simulink model "DKver1"  (R2013b)
settings: Solver=ode45  StartTime=0.0  StopTime=20000.0  RelTol=1e-3
libraries: xbsIndex_r4 x132, dspsrcs4 x4
settings Model: Creator=Robot  LastModifiedBy=Robot32-VM

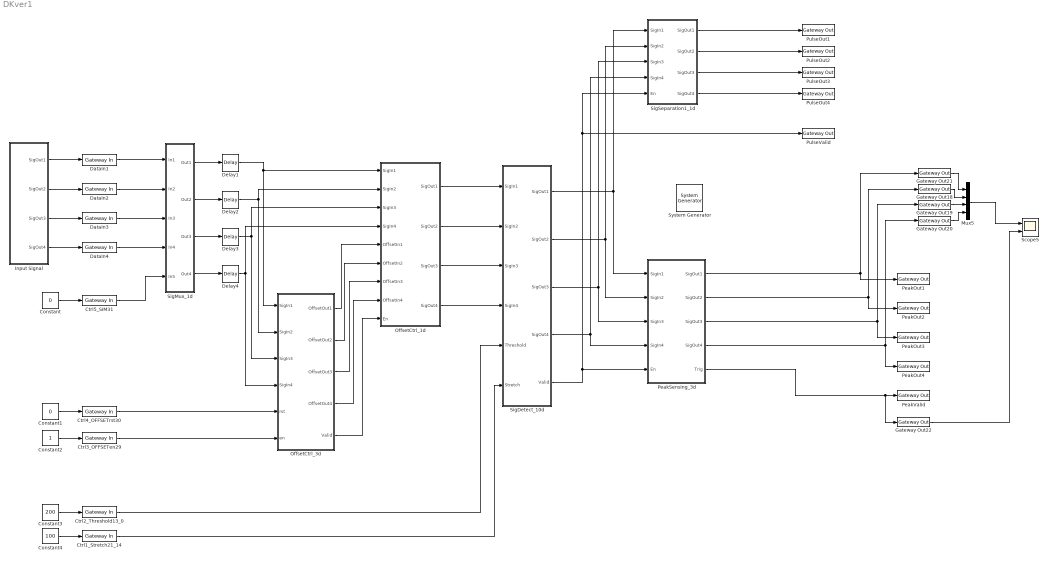
== system DKver1 ==
  " System Generator" : xbsIndex_r4/ System Generator  Tag=genX  xilinxfamily=spartan6  part=xc6slx45  speed=-2  package=fgg484  synthesis_tool=XST  clock_wrapper=Clock Enables  directory=C:/Users/Robot32-VM/Documents/System Generator/11_Gamma_Simple/1_HDL_Netlist_lx45  proj_type=Project Navigator  Synth_file=XST Defaults  Impl_file=ISE Defaults  testbench=off  simulink_period=1  sysclk_period=9  dcm_input_clock_period=10  incr_netlist=off  trim_vbits=Everywhere in SubSystem  dbl_ovrd=According to Block Masks  core_generation=According to Block Masks  run_coregen=off  deprecated_control=off  eval_field=0  block_type=sysgen
  Constant : Constant  Value=0
  Constant1 : Constant  Value=0
  Constant2 : Constant
  Constant3 : Constant  Value=200
  Constant4 : Constant  Value=100
  Ctrl1_Stretch21_14 : xbsIndex_r4/Gateway In  gui_display_data_type=Fixed-point  arith_type=Unsigned  n_bits=8  bin_pt=0  preci_type=Single  exp_width=8  frac_width=24  quantization="Round  (unbiased: +/- Inf)"  overflow=Saturate  period=1  dbl_ovrd=off  timing_constraint=None  locs_specified=off  LOCs={}  UseAsADC=off  ADCChannel='1'  inherit_from_input=off  hdl_port=on  block_type=gatewayin
  Ctrl2_Threshold13_0 : xbsIndex_r4/Gateway In  gui_display_data_type=Fixed-point  arith_type="Signed  (2's comp)"  n_bits=14  bin_pt=0  preci_type=Single  exp_width=8  frac_width=24  quantization="Round  (unbiased: +/- Inf)"  overflow=Saturate  period=1  dbl_ovrd=off  timing_constraint=None  locs_specified=off  LOCs={}  UseAsADC=off  ADCChannel='1'  inherit_from_input=off  hdl_port=on  block_type=gatewayin
  Ctrl3_OFFSETen29 : xbsIndex_r4/Gateway In  gui_display_data_type=Boolean  arith_type=Boolean  n_bits=16  bin_pt=14  preci_type=Single  exp_width=8  frac_width=24  quantization="Round  (unbiased: +/- Inf)"  overflow=Saturate  period=1  dbl_ovrd=off  timing_constraint=None  locs_specified=off  LOCs={}  UseAsADC=off  ADCChannel='1'  inherit_from_input=off  hdl_port=on  block_type=gatewayin
  Ctrl4_OFFSETrst30 : xbsIndex_r4/Gateway In  gui_display_data_type=Boolean  arith_type=Boolean  n_bits=16  bin_pt=14  preci_type=Single  exp_width=8  frac_width=24  quantization="Round  (unbiased: +/- Inf)"  overflow=Saturate  period=1  dbl_ovrd=off  timing_constraint=None  locs_specified=off  LOCs={}  UseAsADC=off  ADCChannel='1'  inherit_from_input=off  hdl_port=on  block_type=gatewayin
  Ctrl5_SIM31 : xbsIndex_r4/Gateway In  gui_display_data_type=Boolean  arith_type=Boolean  n_bits=16  bin_pt=14  preci_type=Single  exp_width=8  frac_width=24  quantization="Round  (unbiased: +/- Inf)"  overflow=Saturate  period=1  dbl_ovrd=off  timing_constraint=None  locs_specified=off  LOCs={}  UseAsADC=off  ADCChannel='1'  inherit_from_input=off  hdl_port=on  block_type=gatewayin
  DataIn{1..4} (4 alike) : xbsIndex_r4/Gateway In  gui_display_data_type=Fixed-point  arith_type="Signed  (2's comp)"  n_bits=14  bin_pt=0  preci_type=Single  exp_width=8  frac_width=24  quantization="Round  (unbiased: +/- Inf)"  overflow=Saturate  period=1  dbl_ovrd=off  timing_constraint=None  locs_specified=off  LOCs={}  UseAsADC=off  ADCChannel='1'  inherit_from_input=off  hdl_port=on  block_type=gatewayin
  Delay{1..4} (4 alike) : xbsIndex_r4/Delay  rst=off  infoeditControl=Selection of Reset will increase slice count due to use of real FFs and instead of SRLs  en=off  latency=1  dbl_ovrd=off  reg_retiming=off  block_type=delay
  Gateway Out{18..22} (5 alike) : xbsIndex_r4/Gateway Out  inherit_from_input=off  hdl_port=off  timing_constraint=None  locs_specified=off  LOCs={}  UseAsDAC=off  DACChannel='1'  block_type=gatewayout
  Input Signal : Subsystem
  Mux5 : Mux
  OffsetCtrl_1d : Subsystem
  OffsetCtrl_3d : Subsystem
  PeakOut{1..4} (4 alike) : xbsIndex_r4/Gateway Out  inherit_from_input=off  hdl_port=on  timing_constraint=None  locs_specified=off  LOCs={}  UseAsDAC=off  DACChannel='1'  block_type=gatewayout
  PeakSensing_3d : Subsystem
  PeakValid : xbsIndex_r4/Gateway Out  inherit_from_input=off  hdl_port=on  timing_constraint=None  locs_specified=off  LOCs={}  UseAsDAC=off  DACChannel='1'  block_type=gatewayout
  PulseOut{1..4} (4 alike) : xbsIndex_r4/Gateway Out  inherit_from_input=off  hdl_port=on  timing_constraint=None  locs_specified=off  LOCs={}  UseAsDAC=off  DACChannel='1'  block_type=gatewayout
  PulseValid : xbsIndex_r4/Gateway Out  inherit_from_input=off  hdl_port=on  timing_constraint=None  locs_specified=off  LOCs={}  UseAsDAC=off  DACChannel='1'  block_type=gatewayout
  Scope5 : Scope  NumInputPorts=2
      settings: YMin=-5~-5  YMax=5~5  SaveName=ScopeData8
  SigDetect_10d : Subsystem
  SigMux_1d : Subsystem
  SigSeparation1_1d : Subsystem
  wires:
  Input Signal/1(SigOut1) -> DataIn1/1
  Input Signal/2(SigOut2) -> DataIn2/1
  Input Signal/3(SigOut3) -> DataIn3/1
  Input Signal/4(SigOut4) -> DataIn4/1
  Constant/1 -> Ctrl5_SIM31/1
  Constant1/1 -> Ctrl4_OFFSETrst30/1
  Constant2/1 -> Ctrl3_OFFSETen29/1
  Constant3/1 -> Ctrl2_Threshold13_0/1
  Constant4/1 -> Ctrl1_Stretch21_14/1
  DataIn1/1 -> SigMux_1d/1(In1)
  DataIn2/1 -> SigMux_1d/2(In2)
  DataIn3/1 -> SigMux_1d/3(In3)
  DataIn4/1 -> SigMux_1d/4(In4)
  Ctrl5_SIM31/1 -> SigMux_1d/5(In5)
  SigMux_1d/1(Out1) -> Delay1/1
  SigMux_1d/2(Out2) -> Delay2/1
  SigMux_1d/3(Out3) -> Delay3/1
  SigMux_1d/4(Out4) -> Delay4/1
  Delay1/1 -> OffsetCtrl_3d/1(SigIn1), OffsetCtrl_1d/1(SigIn1)
  Delay2/1 -> OffsetCtrl_3d/2(SigIn2), OffsetCtrl_1d/2(SigIn2)
  Delay3/1 -> OffsetCtrl_1d/3(SigIn3), OffsetCtrl_3d/3(SigIn3)
  Delay4/1 -> OffsetCtrl_1d/4(SigIn4), OffsetCtrl_3d/4(SigIn4)
  Ctrl4_OFFSETrst30/1 -> OffsetCtrl_3d/5(rst)
  Ctrl3_OFFSETen29/1 -> OffsetCtrl_3d/6(en)
  OffsetCtrl_3d/1(OffsetOut1) -> OffsetCtrl_1d/5(OffsetIn1)
  OffsetCtrl_3d/2(OffsetOut2) -> OffsetCtrl_1d/6(OffsetIn2)
  OffsetCtrl_3d/3(OffsetOut3) -> OffsetCtrl_1d/7(OffsetIn3)
  OffsetCtrl_3d/4(OffsetOut4) -> OffsetCtrl_1d/8(OffsetIn4)
  OffsetCtrl_3d/5(Valid) -> OffsetCtrl_1d/9(En)
  OffsetCtrl_1d/1(SigOut1) -> SigDetect_10d/1(SigIn1)
  OffsetCtrl_1d/2(SigOut2) -> SigDetect_10d/2(SigIn2)
  OffsetCtrl_1d/3(SigOut3) -> SigDetect_10d/3(SigIn3)
  OffsetCtrl_1d/4(SigOut4) -> SigDetect_10d/4(SigIn4)
  Ctrl2_Threshold13_0/1 -> SigDetect_10d/5(Threshold)
  Ctrl1_Stretch21_14/1 -> SigDetect_10d/6(Stretch)
  SigSeparation1_1d/1(SigOut1) -> PulseOut1/1
  SigSeparation1_1d/2(SigOut2) -> PulseOut2/1
  SigSeparation1_1d/3(SigOut3) -> PulseOut3/1
  SigSeparation1_1d/4(SigOut4) -> PulseOut4/1
  SigDetect_10d/1(SigOut1) -> PeakSensing_3d/1(SigIn1), SigSeparation1_1d/1(SigIn1)
  SigDetect_10d/2(SigOut2) -> PeakSensing_3d/2(SigIn2), SigSeparation1_1d/2(SigIn2)
  SigDetect_10d/3(SigOut3) -> PeakSensing_3d/3(SigIn3), SigSeparation1_1d/3(SigIn3)
  SigDetect_10d/4(SigOut4) -> PeakSensing_3d/4(SigIn4), SigSeparation1_1d/4(SigIn4)
  PeakSensing_3d/5(Trig) -> Gateway Out22/1, PeakValid/1
  Mux5/1 -> Scope5/1
  Gateway Out21/1 -> Mux5/1
  Gateway Out18/1 -> Mux5/2
  Gateway Out19/1 -> Mux5/3
  Gateway Out20/1 -> Mux5/4
  Gateway Out22/1 -> Scope5/2
  PeakSensing_3d/1(SigOut1) -> PeakOut1/1, Gateway Out21/1
  PeakSensing_3d/2(SigOut2) -> PeakOut2/1, Gateway Out18/1
  PeakSensing_3d/3(SigOut3) -> PeakOut3/1, Gateway Out19/1
  PeakSensing_3d/4(SigOut4) -> PeakOut4/1, Gateway Out20/1
  SigDetect_10d/5(Valid) -> PulseValid/1, SigSeparation1_1d/5(En), PeakSensing_3d/5(En)

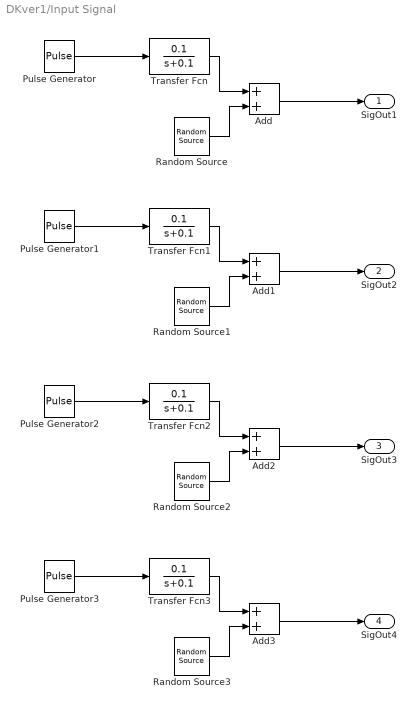
== system DKver1/Input Signal ==
  Add{,1..3} (4 alike) : Sum
  Pulse Generator : DiscretePulseGenerator  PulseType=Time based  Amplitude=5000  Period=1000
  Pulse Generator1 : DiscretePulseGenerator  PulseType=Time based  Amplitude=3000  Period=1000  PulseWidth=2  PhaseDelay=2
  Pulse Generator2 : DiscretePulseGenerator  PulseType=Time based  Amplitude=1000  Period=1000  PulseWidth=2  PhaseDelay=4
  Pulse Generator3 : DiscretePulseGenerator  PulseType=Time based  Amplitude=800  Period=1000  PulseWidth=2  PhaseDelay=6
  Random Source{,1..3} (4 alike) : dspsrcs4/Random Source  SrcType=Uniform  NormMethod=Ziggurat  CltLength=12  MinVal=-100  MaxVal=100  MeanVal=0  VarVal=1  RepMode=Not repeatable  rawSeed=1  IsInherit=off  SampMode=Discrete  SampTime=1  SampFrame=1  DataType=Double  OutComplex=Real
  Transfer Fcn{,1..3} (4 alike) : TransferFcn  Numerator=[0.1]  Denominator=[1 0.1]
  SigOut1 : Outport
  SigOut2 : Outport  Port=2
  SigOut3 : Outport  Port=3
  SigOut4 : Outport  Port=4
  wires:
  Add2/1 -> SigOut3/1
  Add1/1 -> SigOut2/1
  Add3/1 -> SigOut4/1
  Add/1 -> SigOut1/1
  Pulse Generator1/1 -> Transfer Fcn1/1
  Random Source/1 -> Add/2
  Transfer Fcn1/1 -> Add1/1
  Transfer Fcn2/1 -> Add2/1
  Random Source2/1 -> Add2/2
  Transfer Fcn3/1 -> Add3/1
  Pulse Generator3/1 -> Transfer Fcn3/1
  Random Source3/1 -> Add3/2
  Random Source1/1 -> Add1/2
  Pulse Generator2/1 -> Transfer Fcn2/1
  Transfer Fcn/1 -> Add/1
  Pulse Generator/1 -> Transfer Fcn/1

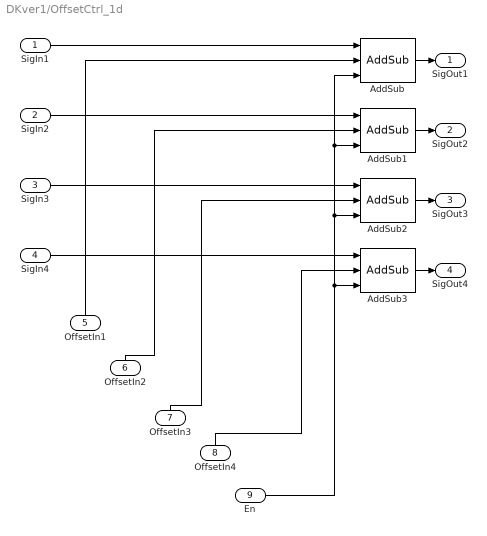
== system DKver1/OffsetCtrl_1d ==
  SigIn1 : Inport
  SigIn2 : Inport  Port=2
  SigIn3 : Inport  Port=3
  SigIn4 : Inport  Port=4
  OffsetIn1 : Inport  Port=5
  OffsetIn2 : Inport  Port=6
  OffsetIn3 : Inport  Port=7
  OffsetIn4 : Inport  Port=8
  En : Inport  Port=9
  AddSub{,1..3} (4 alike) : xbsIndex_r4/AddSub  mode=Subtraction  use_carryin=off  use_carryout=off  en=on  latency=1  precision=User Defined  arith_type="Signed  (2's comp)"  n_bits=14  bin_pt=0  quantization="Round  (unbiased: +/- Inf)"  overflow=Saturate  dbl_ovrd=off  use_behavioral_HDL=off  hw_selection=Fabric  pipelined=off  block_type=addsub
  SigOut1 : Outport
  SigOut2 : Outport  Port=2
  SigOut3 : Outport  Port=3
  SigOut4 : Outport  Port=4
  wires:
  OffsetIn1/1 -> AddSub/2
  SigIn4/1 -> AddSub3/1
  AddSub3/1 -> SigOut4/1
  En/1 -> AddSub3/3, AddSub2/3, AddSub1/3, AddSub/3
  SigIn2/1 -> AddSub1/1
  AddSub/1 -> SigOut1/1
  OffsetIn3/1 -> AddSub2/2
  AddSub1/1 -> SigOut2/1
  OffsetIn4/1 -> AddSub3/2
  AddSub2/1 -> SigOut3/1
  SigIn3/1 -> AddSub2/1
  SigIn1/1 -> AddSub/1
  OffsetIn2/1 -> AddSub1/2

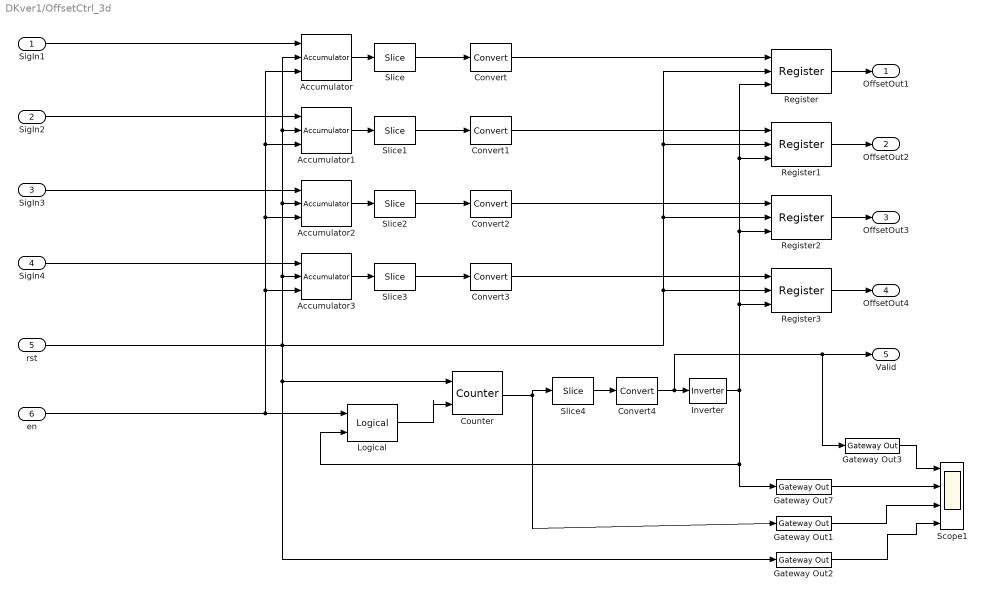
== system DKver1/OffsetCtrl_3d ==
  SigIn1 : Inport
  SigIn2 : Inport  Port=2
  SigIn3 : Inport  Port=3
  SigIn4 : Inport  Port=4
  rst : Inport  Port=5
  en : Inport  Port=6
  Accumulator{,1..3} (4 alike) : xbsIndex_r4/Accumulator  operation=Add  n_bits=32  overflow=Wrap  scale=1  rst=on  infoeditControl=reset for floating point data type must be asserted for a minimum of 2 cycles  hasbypass=off  en=on  latency=0  dbl_ovrd=off  msb_inp=100  msb=100  lsb=-100  use_behavioral_HDL=on  implementation=Fabric  block_type=accum
  Convert{,1..3} (4 alike) : xbsIndex_r4/Convert  gui_display_data_type=Fixed-point  arith_type="Signed  (2's comp)"  n_bits=20  bin_pt=0  float_type=Single  exp_bits=8  fraction_bits=24  quantization="Round  (unbiased: +/- Inf)"  overflow=Wrap  en=off  latency=1  dbl_ovrd=off  pipeline=off  block_type=convert
  Convert4 : xbsIndex_r4/Convert  gui_display_data_type=Boolean  arith_type=Boolean  n_bits=20  bin_pt=0  float_type=Single  exp_bits=8  fraction_bits=24  quantization="Round  (unbiased: +/- Inf)"  overflow=Wrap  en=off  latency=1  dbl_ovrd=off  pipeline=off  block_type=convert
  Counter : xbsIndex_r4/Counter  cnt_type=Free Running  cnt_to=4000  operation=Up  start_count=0  cnt_by_val=1  arith_type=Unsigned  n_bits=13  bin_pt=0  load_pin=off  rst=on  en=on  explicit_period=on  period=1  dbl_ovrd=off  use_behavioral_HDL=off  implementation=Fabric  block_type=counter
  Gateway Out{1..3,7} (4 alike) : xbsIndex_r4/Gateway Out  inherit_from_input=off  hdl_port=off  timing_constraint=None  locs_specified=off  LOCs={}  UseAsDAC=off  DACChannel='1'  block_type=gatewayout
  Inverter : xbsIndex_r4/Inverter  en=off  latency=1  dbl_ovrd=off  block_type=inv
  Logical : xbsIndex_r4/Logical  logical_function=AND  inputs=2  en=off  latency=1  precision=Full  arith_type=Unsigned  n_bits=16  bin_pt=0  align_bp=on  dbl_ovrd=off  block_type=logical
  Register{,1..3} (4 alike) : xbsIndex_r4/Register  init=0  rst=on  en=on  dbl_ovrd=off  block_type=register
  Scope1 : Scope  NumInputPorts=4
      settings: YMin=-5~-5~-5~-5  YMax=5~5~5~5
  Slice{,1..3} (4 alike) : xbsIndex_r4/Slice  nbits=20  boolean_output=off  mode=Upper Bit Location + Width  bit1=0  base1=MSB of Input  bit0=0  base0=LSB of Input  dbl_ovrd=off  block_type=slice
  Slice4 : xbsIndex_r4/Slice  nbits=1  boolean_output=off  mode=Upper Bit Location + Width  bit1=0  base1=MSB of Input  bit0=0  base0=LSB of Input  dbl_ovrd=off  block_type=slice
  OffsetOut1 : Outport
  OffsetOut2 : Outport  Port=2
  OffsetOut3 : Outport  Port=3
  OffsetOut4 : Outport  Port=4
  Valid : Outport  Port=5
  wires:
  Accumulator/1 -> Slice/1
  Accumulator1/1 -> Slice1/1
  Accumulator2/1 -> Slice2/1
  Accumulator3/1 -> Slice3/1
  Slice/1 -> Convert/1
  Slice1/1 -> Convert1/1
  Slice2/1 -> Convert2/1
  Slice3/1 -> Convert3/1
  Convert/1 -> Register/1
  Convert1/1 -> Register1/1
  Convert2/1 -> Register2/1
  Convert3/1 -> Register3/1
  Register/1 -> OffsetOut1/1
  Register1/1 -> OffsetOut2/1
  Register2/1 -> OffsetOut3/1
  Register3/1 -> OffsetOut4/1
  rst/1 -> Accumulator/2, Accumulator1/2, Accumulator2/2, Accumulator3/2, Register3/2, Register2/2, Register1/2, Register/2, Gateway Out2/1, Counter/1
  Gateway Out7/1 -> Scope1/2
  Counter/1 -> Gateway Out1/1, Slice4/1
  Slice4/1 -> Convert4/1
  Gateway Out1/1 -> Scope1/3
  Logical/1 -> Counter/2
  Gateway Out2/1 -> Scope1/4
  en/1 -> Accumulator/3, Accumulator1/3, Accumulator2/3, Accumulator3/3, Logical/1
  SigIn1/1 -> Accumulator/1
  SigIn2/1 -> Accumulator1/1
  SigIn3/1 -> Accumulator2/1
  SigIn4/1 -> Accumulator3/1
  Convert4/1 -> Gateway Out3/1, Valid/1, Inverter/1
  Inverter/1 -> Register/3, Register1/3, Register2/3, Register3/3, Logical/2, Gateway Out7/1
  Gateway Out3/1 -> Scope1/1

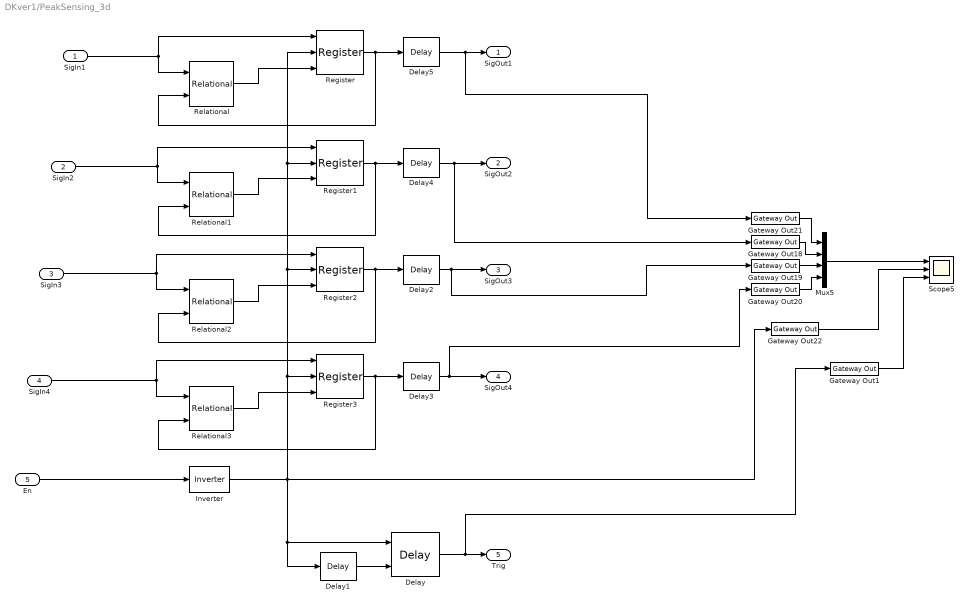
== system DKver1/PeakSensing_3d ==
  SigIn1 : Inport
  SigIn2 : Inport  Port=2
  SigIn3 : Inport  Port=3
  SigIn4 : Inport  Port=4
  En : Inport  Port=5
  Delay : xbsIndex_r4/Delay  rst=on  infoeditControl=Selection of Reset will increase slice count due to use of real FFs and instead of SRLs  en=off  latency=1  dbl_ovrd=off  reg_retiming=off  block_type=delay
  Delay1 : xbsIndex_r4/Delay  rst=off  infoeditControl=Selection of Reset will increase slice count due to use of real FFs and instead of SRLs  en=off  latency=1  dbl_ovrd=off  reg_retiming=off  block_type=delay
  Delay{2..5} (4 alike) : xbsIndex_r4/Delay  rst=off  infoeditControl=Selection of Reset will increase slice count due to use of real FFs and instead of SRLs  en=off  latency=2  dbl_ovrd=off  reg_retiming=off  block_type=delay
  Gateway Out{1,18..22} (6 alike) : xbsIndex_r4/Gateway Out  inherit_from_input=off  hdl_port=off  timing_constraint=None  locs_specified=off  LOCs={}  UseAsDAC=off  DACChannel='1'  block_type=gatewayout
  Inverter : xbsIndex_r4/Inverter  en=off  latency=1  dbl_ovrd=off  block_type=inv
  Mux5 : Mux
  Register{,1..3} (4 alike) : xbsIndex_r4/Register  init=0  rst=on  en=on  dbl_ovrd=off  block_type=register
  Relational{,1..3} (4 alike) : xbsIndex_r4/Relational  mode=a>b  en=off  latency=0  dbl_ovrd=off  block_type=relational
  Scope5 : Scope  NumInputPorts=3
      settings: YMin=-5~-5~-5  YMax=5~5~5  SaveName=ScopeData7
  SigOut1 : Outport
  SigOut2 : Outport  Port=2
  SigOut3 : Outport  Port=3
  SigOut4 : Outport  Port=4
  Trig : Outport  Port=5
  wires:
  Relational3/1 -> Register3/3
  Register3/1 -> Delay3/1, Relational3/2
  Register/1 -> Relational/2, Delay5/1
  Relational/1 -> Register/3
  Relational1/1 -> Register1/3
  Register1/1 -> Delay4/1, Relational1/2
  Relational2/1 -> Register2/3
  Register2/1 -> Delay2/1, Relational2/2
  Inverter/1 -> Delay1/1, Delay/1, Register/2, Register1/2, Register2/2, Register3/2, Gateway Out22/1
  Mux5/1 -> Scope5/1
  Gateway Out21/1 -> Mux5/1
  Gateway Out18/1 -> Mux5/2
  Gateway Out19/1 -> Mux5/3
  Gateway Out20/1 -> Mux5/4
  Gateway Out22/1 -> Scope5/2
  En/1 -> Inverter/1
  SigIn1/1 -> Register/1, Relational/1
  SigIn4/1 -> Register3/1, Relational3/1
  SigIn2/1 -> Register1/1, Relational1/1
  SigIn3/1 -> Register2/1, Relational2/1
  Delay1/1 -> Delay/2
  Delay/1 -> Gateway Out1/1, Trig/1
  Gateway Out1/1 -> Scope5/3
  Delay3/1 -> SigOut4/1, Gateway Out20/1
  Delay2/1 -> Gateway Out19/1, SigOut3/1
  Delay4/1 -> Gateway Out18/1, SigOut2/1
  Delay5/1 -> Gateway Out21/1, SigOut1/1

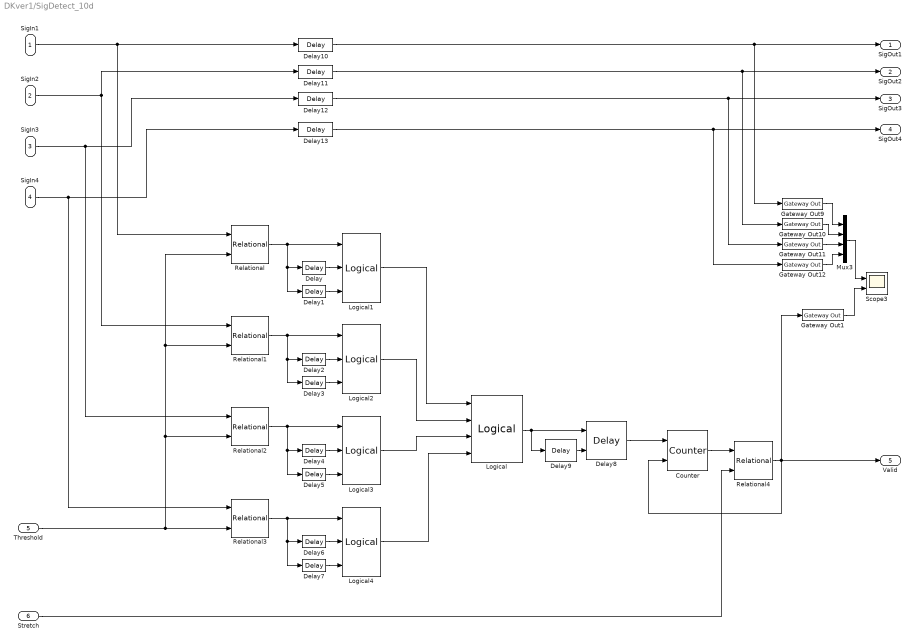
== system DKver1/SigDetect_10d ==
  SigIn1 : Inport
  SigIn2 : Inport  Port=2
  SigIn3 : Inport  Port=3
  SigIn4 : Inport  Port=4
  Threshold : Inport  Port=5
  Stretch : Inport  Port=6
  Counter : xbsIndex_r4/Counter  cnt_type=Free Running  cnt_to=Inf  operation=Up  start_count=0  cnt_by_val=1  arith_type=Unsigned  n_bits=32  bin_pt=0  load_pin=off  rst=on  en=on  explicit_period=on  period=1  dbl_ovrd=off  use_behavioral_HDL=off  implementation=Fabric  block_type=counter
  Delay{,2,4,6,9} (5 alike) : xbsIndex_r4/Delay  rst=off  infoeditControl=Selection of Reset will increase slice count due to use of real FFs and instead of SRLs  en=off  latency=1  dbl_ovrd=off  reg_retiming=off  block_type=delay
  Delay{1,3,5,7} (4 alike) : xbsIndex_r4/Delay  rst=off  infoeditControl=Selection of Reset will increase slice count due to use of real FFs and instead of SRLs  en=off  latency=2  dbl_ovrd=off  reg_retiming=off  block_type=delay
  Delay{10..13} (4 alike) : xbsIndex_r4/Delay  rst=off  infoeditControl=Selection of Reset will increase slice count due to use of real FFs and instead of SRLs  en=off  latency=10  dbl_ovrd=off  reg_retiming=off  block_type=delay
  Delay8 : xbsIndex_r4/Delay  rst=on  infoeditControl=Selection of Reset will increase slice count due to use of real FFs and instead of SRLs  en=off  latency=1  dbl_ovrd=off  reg_retiming=off  block_type=delay
  Gateway Out{1,9..12} (5 alike) : xbsIndex_r4/Gateway Out  inherit_from_input=off  hdl_port=off  timing_constraint=None  locs_specified=off  LOCs={}  UseAsDAC=off  DACChannel='1'  block_type=gatewayout
  Logical : xbsIndex_r4/Logical  logical_function=OR  inputs=4  en=off  latency=0  precision=Full  arith_type=Unsigned  n_bits=16  bin_pt=0  align_bp=on  dbl_ovrd=off  block_type=logical
  Logical{1..4} (4 alike) : xbsIndex_r4/Logical  logical_function=AND  inputs=3  en=off  latency=0  precision=Full  arith_type=Unsigned  n_bits=16  bin_pt=0  align_bp=on  dbl_ovrd=off  block_type=logical
  Mux3 : Mux
  Relational{,1..3} (4 alike) : xbsIndex_r4/Relational  mode=a>b  en=off  latency=1  dbl_ovrd=off  block_type=relational
  Relational4 : xbsIndex_r4/Relational  mode=a<b  en=off  latency=1  dbl_ovrd=off  block_type=relational
  Scope3 : Scope  NumInputPorts=2
      settings: YMin=-5~-5  YMax=5~5  SaveName=ScopeData4
  SigOut1 : Outport
  SigOut2 : Outport  Port=2
  SigOut3 : Outport  Port=3
  SigOut4 : Outport  Port=4
  Valid : Outport  Port=5
  wires:
  SigIn2/1 -> Relational1/1, Delay11/1
  SigIn1/1 -> Relational/1, Delay10/1
  Threshold/1 -> Relational/2, Relational1/2, Relational2/2, Relational3/2
  SigIn4/1 -> Delay13/1, Relational3/1
  SigIn3/1 -> Delay12/1, Relational2/1
  Relational/1 -> Delay1/1, Delay/1, Logical1/1
  Delay/1 -> Logical1/2
  Delay1/1 -> Logical1/3
  Relational1/1 -> Logical2/1, Delay2/1, Delay3/1
  Delay2/1 -> Logical2/2
  Delay3/1 -> Logical2/3
  Relational2/1 -> Delay5/1, Delay4/1, Logical3/1
  Delay4/1 -> Logical3/2
  Delay5/1 -> Logical3/3
  Relational3/1 -> Logical4/1, Delay6/1, Delay7/1
  Delay6/1 -> Logical4/2
  Delay7/1 -> Logical4/3
  Logical1/1 -> Logical/1
  Logical2/1 -> Logical/2
  Logical3/1 -> Logical/3
  Logical4/1 -> Logical/4
  Logical/1 -> Delay9/1, Delay8/1
  Delay9/1 -> Delay8/2
  Delay8/1 -> Counter/1
  Counter/1 -> Relational4/1
  Stretch/1 -> Relational4/2
  Relational4/1 -> Valid/1, Counter/2, Gateway Out1/1
  Mux3/1 -> Scope3/1
  Gateway Out9/1 -> Mux3/1
  Gateway Out10/1 -> Mux3/2
  Gateway Out11/1 -> Mux3/3
  Gateway Out12/1 -> Mux3/4
  Gateway Out1/1 -> Scope3/2
  Delay10/1 -> Gateway Out9/1, SigOut1/1
  Delay11/1 -> Gateway Out10/1, SigOut2/1
  Delay12/1 -> Gateway Out11/1, SigOut3/1
  Delay13/1 -> Gateway Out12/1, SigOut4/1

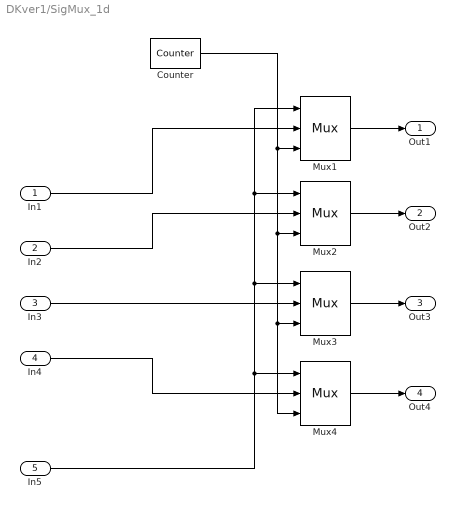
== system DKver1/SigMux_1d ==
  In1 : Inport
  In2 : Inport  Port=2
  In3 : Inport  Port=3
  In4 : Inport  Port=4
  In5 : Inport  Port=5
  Counter : xbsIndex_r4/Counter  cnt_type=Free Running  cnt_to=Inf  operation=Up  start_count=0  cnt_by_val=1  arith_type="Signed  (2's comp)"  n_bits=11  bin_pt=0  load_pin=off  rst=off  en=off  explicit_period=on  period=1  dbl_ovrd=off  use_behavioral_HDL=off  implementation=Fabric  block_type=counter
  Mux{1..4} (4 alike) : xbsIndex_r4/Mux  inputs=2  en=off  latency=1  precision=Full  arith_type=Unsigned  n_bits=16  bin_pt=14  quantization=Truncate  overflow=Wrap  dbl_ovrd=off  block_type=mux
  Out1 : Outport
  Out2 : Outport  Port=2
  Out3 : Outport  Port=3
  Out4 : Outport  Port=4
  wires:
  Mux4/1 -> Out4/1
  Mux3/1 -> Out3/1
  Mux2/1 -> Out2/1
  Mux1/1 -> Out1/1
  Counter/1 -> Mux4/3, Mux3/3, Mux2/3, Mux1/3
  In5/1 -> Mux4/1, Mux3/1, Mux2/1, Mux1/1
  In3/1 -> Mux3/2
  In2/1 -> Mux2/2
  In1/1 -> Mux1/2
  In4/1 -> Mux4/2

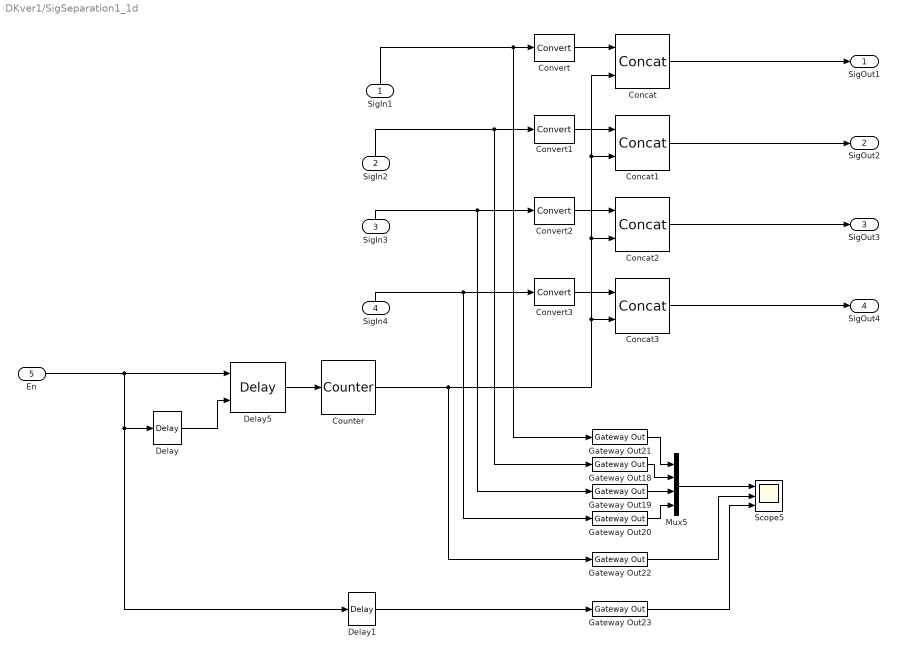
== system DKver1/SigSeparation1_1d ==
  SigIn1 : Inport
  SigIn2 : Inport  Port=2
  SigIn3 : Inport  Port=3
  SigIn4 : Inport  Port=4
  En : Inport  Port=5
  Concat{,1..3} (4 alike) : xbsIndex_r4/Concat  num_inputs=2  dbl_ovrd=off  block_type=concat
  Convert{,1..3} (4 alike) : xbsIndex_r4/Convert  gui_display_data_type=Fixed-point  arith_type=Unsigned  n_bits=14  bin_pt=0  float_type=Single  exp_bits=8  fraction_bits=24  quantization="Round  (unbiased: +/- Inf)"  overflow=Wrap  en=off  latency=1  dbl_ovrd=off  pipeline=off  block_type=convert
  Counter : xbsIndex_r4/Counter  cnt_type=Free Running  cnt_to=Inf  operation=Up  start_count=0  cnt_by_val=1  arith_type=Unsigned  n_bits=2  bin_pt=0  load_pin=off  rst=off  en=on  explicit_period=on  period=1  dbl_ovrd=off  use_behavioral_HDL=off  implementation=Fabric  block_type=counter
  Delay : xbsIndex_r4/Delay  rst=off  infoeditControl=Selection of Reset will increase slice count due to use of real FFs and instead of SRLs  en=off  latency=1  dbl_ovrd=off  reg_retiming=off  block_type=delay
  Delay1 : xbsIndex_r4/Delay  rst=off  infoeditControl=Selection of Reset will increase slice count due to use of real FFs and instead of SRLs  en=off  latency=0  dbl_ovrd=off  reg_retiming=off  block_type=delay
  Delay5 : xbsIndex_r4/Delay  rst=on  infoeditControl=Selection of Reset will increase slice count due to use of real FFs and instead of SRLs  en=off  latency=1  dbl_ovrd=off  reg_retiming=off  block_type=delay
  Gateway Out{18..23} (6 alike) : xbsIndex_r4/Gateway Out  inherit_from_input=off  hdl_port=off  timing_constraint=None  locs_specified=off  LOCs={}  UseAsDAC=off  DACChannel='1'  block_type=gatewayout
  Mux5 : Mux
  Scope5 : Scope  NumInputPorts=3
      settings: YMin=-5~-5~-5  YMax=5~5~5  SaveName=ScopeData6
  SigOut1 : Outport
  SigOut2 : Outport  Port=2
  SigOut3 : Outport  Port=3
  SigOut4 : Outport  Port=4
  wires:
  Concat2/1 -> SigOut3/1
  Concat1/1 -> SigOut2/1
  Concat3/1 -> SigOut4/1
  Concat/1 -> SigOut1/1
  Delay/1 -> Delay5/2
  Convert3/1 -> Concat3/1
  Convert1/1 -> Concat1/1
  Convert2/1 -> Concat2/1
  Convert/1 -> Concat/1
  Delay5/1 -> Counter/1
  SigIn3/1 -> Gateway Out19/1, Convert2/1
  SigIn2/1 -> Gateway Out18/1, Convert1/1
  SigIn1/1 -> Gateway Out21/1, Convert/1
  SigIn4/1 -> Gateway Out20/1, Convert3/1
  En/1 -> Delay1/1, Delay/1, Delay5/1
  Gateway Out23/1 -> Scope5/3
  Counter/1 -> Gateway Out22/1, Concat/2, Concat1/2, Concat2/2, Concat3/2
  Mux5/1 -> Scope5/1
  Gateway Out21/1 -> Mux5/1
  Gateway Out18/1 -> Mux5/2
  Gateway Out19/1 -> Mux5/3
  Gateway Out20/1 -> Mux5/4
  Gateway Out22/1 -> Scope5/2
  Delay1/1 -> Gateway Out23/1
